simulink model "motorStyrning"  (R2020b)
settings: Solver=VariableStepAuto  StartTime=0.0  StopTime=0.1  RelTol=1e-3
model workspace (MAT data in the model file):
  intervall = 300
  intervall2 = 1
  intervall3 = 1
  timeTTT : Simulink.Signal (value not decoded)
libraries: fl_lib x116, ee_lib x24, nesl_utility x23
(part 2 of 2)

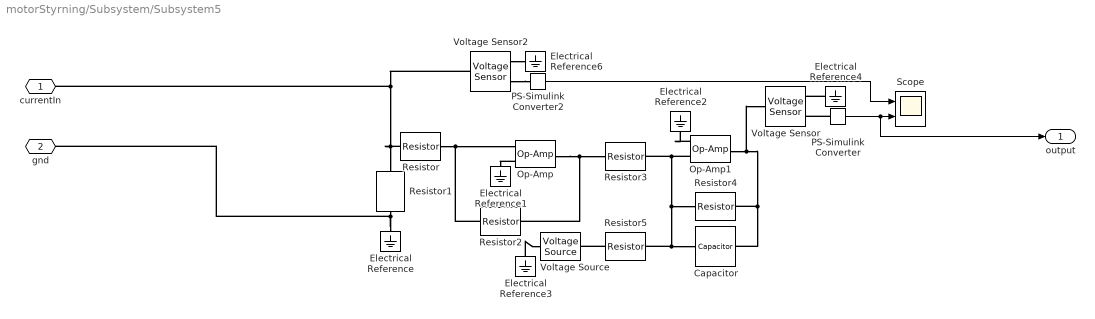
== system motorStyrning/Subsystem/Subsystem5 ==
  Capacitor : fl_lib/Electrical/Electrical Elements/Capacitor  c=10 nF  r=1e-6 Ohm  g=0 1/Ohm  i_specify=off  i_priority=None  i=0 A  i_nominal_specify=off  i_nominal_unit=A  i_nominal_value=1  v_specify=off  v_priority=None  v=0 V  v_nominal_specify=off  v_nominal_unit=V  v_nominal_value=1  vc_specify=off  vc_priority=High  vc=0 V  vc_nominal_specify=off  vc_nominal_unit=V  vc_nominal_value=1
  Electrical Reference{,1..4,6} (6 alike) : fl_lib/Electrical/Electrical Elements/Electrical Reference
  Op-Amp : fl_lib/Electrical/Electrical Elements/Op-Amp  outI_specify=off  outI_priority=None  outI=0 A  outI_nominal_specify=off  outI_nominal_unit=A  outI_nominal_value=1
  Op-Amp1 : fl_lib/Electrical/Electrical Elements/Op-Amp  outI_specify=off  outI_priority=None  outI=0 A  outI_nominal_specify=off  outI_nominal_unit=A  outI_nominal_value=1
  PS-Simulink Converter : nesl_utility/PS-Simulink Converter  PhysicalDomain=network_engine_domain  SubClassName=ps_output  LeftPortType=input  RightPortType=output  PseudoPeriodic=off  Frequencies=[]  Unit=inherit  AffineConversion=off
  PS-Simulink Converter2 : nesl_utility/PS-Simulink Converter  PhysicalDomain=network_engine_domain  SubClassName=ps_output  LeftPortType=input  RightPortType=output  PseudoPeriodic=off  Frequencies=[]  Unit=inherit  AffineConversion=off
  Resistor : fl_lib/Electrical/Electrical Elements/Resistor  R=10 kOhm  i_specify=off  i_priority=None  i=0 A  i_nominal_specify=off  i_nominal_unit=A  i_nominal_value=1  v_specify=off  v_priority=None  v=0 V  v_nominal_specify=off  v_nominal_unit=V  v_nominal_value=1
  Resistor1 : fl_lib/Electrical/Electrical Elements/Resistor  R=60 Ohm  i_specify=off  i_priority=None  i=0 A  i_nominal_specify=off  i_nominal_unit=A  i_nominal_value=1  v_specify=off  v_priority=None  v=0 V  v_nominal_specify=off  v_nominal_unit=V  v_nominal_value=1
  Resistor2 : fl_lib/Electrical/Electrical Elements/Resistor  R=8275 Ohm  i_specify=off  i_priority=None  i=0 A  i_nominal_specify=off  i_nominal_unit=A  i_nominal_value=1  v_specify=off  v_priority=None  v=0 V  v_nominal_specify=off  v_nominal_unit=V  v_nominal_value=1
  Resistor3 : fl_lib/Electrical/Electrical Elements/Resistor  R=10 kOhm  i_specify=off  i_priority=None  i=0 A  i_nominal_specify=off  i_nominal_unit=A  i_nominal_value=1  v_specify=off  v_priority=None  v=0 V  v_nominal_specify=off  v_nominal_unit=V  v_nominal_value=1
  Resistor4 : fl_lib/Electrical/Electrical Elements/Resistor  R=10 kOhm  i_specify=off  i_priority=None  i=0 A  i_nominal_specify=off  i_nominal_unit=A  i_nominal_value=1  v_specify=off  v_priority=None  v=0 V  v_nominal_specify=off  v_nominal_unit=V  v_nominal_value=1
  Resistor5 : fl_lib/Electrical/Electrical Elements/Resistor  R=29.7 kOhm  i_specify=off  i_priority=None  i=0 A  i_nominal_specify=off  i_nominal_unit=A  i_nominal_value=1  v_specify=off  v_priority=None  v=0 V  v_nominal_specify=off  v_nominal_unit=V  v_nominal_value=1
  Scope : Scope  NumInputPorts=2
  Voltage Sensor : fl_lib/Electrical/Electrical Sensors/Voltage Sensor
  Voltage Sensor2 : fl_lib/Electrical/Electrical Sensors/Voltage Sensor
  Voltage Source : ee_lib/Sources/Voltage Source  dc_voltage=-15 V  ac_voltage=0 V  ac_shift=0 rad  ac_frequency=60 Hz  noise_mode=0  PSD=0 V^2/Hz  repeatability=1  auto_seed=3243031446  user_seed=0  sample_time=1e-3 s  i_specify=off  i_priority=None  i=0 A  i_nominal_specify=off  i_nominal_unit=A  i_nominal_value=1  v_specify=off  v_priority=None  v=0 V  v_nominal_specify=off  v_nominal_unit=V  v_nominal_value=1
  currentIn : PMIOPort  Side=Left
  gnd : PMIOPort  Port=2  Side=Left
  output : Outport
  wires:
  PS-Simulink Converter/1 -> output/1, Scope/2
  PS-Simulink Converter2/1 -> Scope/1
  connections:
  Resistor1/RConn1 -- gnd/RConn1 -- Electrical Reference/LConn1
  Voltage Sensor2/RConn1 -- PS-Simulink Converter2/LConn1
  Voltage Sensor2/RConn2 -- Electrical Reference6/LConn1
  PS-Simulink Converter/LConn1 -- Voltage Sensor/RConn1
  Resistor5/LConn1 -- Voltage Source/LConn1
  Op-Amp/LConn2 -- Electrical Reference1/LConn1
  Op-Amp1/LConn2 -- Resistor3/RConn1 -- Resistor5/RConn1 -- Capacitor/LConn1 -- Resistor4/LConn1
  Electrical Reference3/LConn1 -- Voltage Source/RConn1
  Electrical Reference4/LConn1 -- Voltage Sensor/RConn2
  Op-Amp1/LConn1 -- Electrical Reference2/LConn1
  Capacitor/RConn1 -- Resistor4/RConn1 -- Op-Amp1/RConn1 -- Voltage Sensor/LConn1
  Op-Amp/RConn1 -- Resistor3/LConn1 -- Resistor2/RConn1
  Resistor/RConn1 -- Resistor2/LConn1 -- Op-Amp/LConn1
  Voltage Sensor2/LConn1 -- Resistor/LConn1 -- Resistor1/LConn1 -- currentIn/RConn1

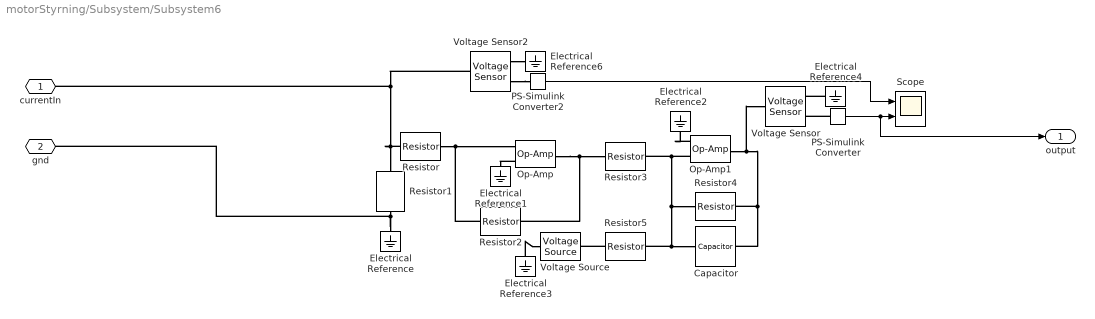
== system motorStyrning/Subsystem/Subsystem6 ==
  Capacitor : fl_lib/Electrical/Electrical Elements/Capacitor  c=10 nF  r=1e-6 Ohm  g=0 1/Ohm  i_specify=off  i_priority=None  i=0 A  i_nominal_specify=off  i_nominal_unit=A  i_nominal_value=1  v_specify=off  v_priority=None  v=0 V  v_nominal_specify=off  v_nominal_unit=V  v_nominal_value=1  vc_specify=off  vc_priority=High  vc=0 V  vc_nominal_specify=off  vc_nominal_unit=V  vc_nominal_value=1
  Electrical Reference{,1..4,6} (6 alike) : fl_lib/Electrical/Electrical Elements/Electrical Reference
  Op-Amp : fl_lib/Electrical/Electrical Elements/Op-Amp  outI_specify=off  outI_priority=None  outI=0 A  outI_nominal_specify=off  outI_nominal_unit=A  outI_nominal_value=1
  Op-Amp1 : fl_lib/Electrical/Electrical Elements/Op-Amp  outI_specify=off  outI_priority=None  outI=0 A  outI_nominal_specify=off  outI_nominal_unit=A  outI_nominal_value=1
  PS-Simulink Converter : nesl_utility/PS-Simulink Converter  PhysicalDomain=network_engine_domain  SubClassName=ps_output  LeftPortType=input  RightPortType=output  PseudoPeriodic=off  Frequencies=[]  Unit=inherit  AffineConversion=off
  PS-Simulink Converter2 : nesl_utility/PS-Simulink Converter  PhysicalDomain=network_engine_domain  SubClassName=ps_output  LeftPortType=input  RightPortType=output  PseudoPeriodic=off  Frequencies=[]  Unit=inherit  AffineConversion=off
  Resistor : fl_lib/Electrical/Electrical Elements/Resistor  R=10 kOhm  i_specify=off  i_priority=None  i=0 A  i_nominal_specify=off  i_nominal_unit=A  i_nominal_value=1  v_specify=off  v_priority=None  v=0 V  v_nominal_specify=off  v_nominal_unit=V  v_nominal_value=1
  Resistor1 : fl_lib/Electrical/Electrical Elements/Resistor  R=60 Ohm  i_specify=off  i_priority=None  i=0 A  i_nominal_specify=off  i_nominal_unit=A  i_nominal_value=1  v_specify=off  v_priority=None  v=0 V  v_nominal_specify=off  v_nominal_unit=V  v_nominal_value=1
  Resistor2 : fl_lib/Electrical/Electrical Elements/Resistor  R=8275 Ohm  i_specify=off  i_priority=None  i=0 A  i_nominal_specify=off  i_nominal_unit=A  i_nominal_value=1  v_specify=off  v_priority=None  v=0 V  v_nominal_specify=off  v_nominal_unit=V  v_nominal_value=1
  Resistor3 : fl_lib/Electrical/Electrical Elements/Resistor  R=10 kOhm  i_specify=off  i_priority=None  i=0 A  i_nominal_specify=off  i_nominal_unit=A  i_nominal_value=1  v_specify=off  v_priority=None  v=0 V  v_nominal_specify=off  v_nominal_unit=V  v_nominal_value=1
  Resistor4 : fl_lib/Electrical/Electrical Elements/Resistor  R=10 kOhm  i_specify=off  i_priority=None  i=0 A  i_nominal_specify=off  i_nominal_unit=A  i_nominal_value=1  v_specify=off  v_priority=None  v=0 V  v_nominal_specify=off  v_nominal_unit=V  v_nominal_value=1
  Resistor5 : fl_lib/Electrical/Electrical Elements/Resistor  R=29.7 kOhm  i_specify=off  i_priority=None  i=0 A  i_nominal_specify=off  i_nominal_unit=A  i_nominal_value=1  v_specify=off  v_priority=None  v=0 V  v_nominal_specify=off  v_nominal_unit=V  v_nominal_value=1
  Scope : Scope  NumInputPorts=2
  Voltage Sensor : fl_lib/Electrical/Electrical Sensors/Voltage Sensor
  Voltage Sensor2 : fl_lib/Electrical/Electrical Sensors/Voltage Sensor
  Voltage Source : ee_lib/Sources/Voltage Source  dc_voltage=-15 V  ac_voltage=0 V  ac_shift=0 rad  ac_frequency=60 Hz  noise_mode=0  PSD=0 V^2/Hz  repeatability=1  auto_seed=4112460543  user_seed=0  sample_time=1e-3 s  i_specify=off  i_priority=None  i=0 A  i_nominal_specify=off  i_nominal_unit=A  i_nominal_value=1  v_specify=off  v_priority=None  v=0 V  v_nominal_specify=off  v_nominal_unit=V  v_nominal_value=1
  currentIn : PMIOPort  Side=Left
  gnd : PMIOPort  Port=2  Side=Left
  output : Outport
  wires:
  PS-Simulink Converter/1 -> output/1, Scope/2
  PS-Simulink Converter2/1 -> Scope/1
  connections:
  Resistor1/RConn1 -- Electrical Reference/LConn1 -- gnd/RConn1
  Voltage Sensor2/RConn1 -- PS-Simulink Converter2/LConn1
  Voltage Sensor2/RConn2 -- Electrical Reference6/LConn1
  PS-Simulink Converter/LConn1 -- Voltage Sensor/RConn1
  Resistor5/LConn1 -- Voltage Source/LConn1
  Op-Amp/LConn2 -- Electrical Reference1/LConn1
  Op-Amp1/LConn2 -- Resistor3/RConn1 -- Resistor5/RConn1 -- Capacitor/LConn1 -- Resistor4/LConn1
  Electrical Reference3/LConn1 -- Voltage Source/RConn1
  Electrical Reference4/LConn1 -- Voltage Sensor/RConn2
  Op-Amp1/LConn1 -- Electrical Reference2/LConn1
  Capacitor/RConn1 -- Resistor4/RConn1 -- Op-Amp1/RConn1 -- Voltage Sensor/LConn1
  Op-Amp/RConn1 -- Resistor3/LConn1 -- Resistor2/RConn1
  Resistor/RConn1 -- Resistor2/LConn1 -- Op-Amp/LConn1
  Voltage Sensor2/LConn1 -- Resistor/LConn1 -- Resistor1/LConn1 -- currentIn/RConn1

== matlab function motorStyrning/Subsystem/MATLAB Function ==
  data: freeW input; u input; y output
function y = fcn(freeW, u)
%#codegen
if u == 2
    
    if freeW==0
    a0 = 0; a1 = 0; a2 = 10; b0 = 10; b1 = 0; b2 = 10;  %% a2 var 10 innan AW ändrade
    else
    a0 = 0; a1 = 0; a2 = 10; b0 = 0; b1 = 0; b2 = 10;   %% a2 var 10 innan AW ändrade
    end
    
elseif u == 10 || 32
    
    if freeW == 0
      a0 = 0; a1 = 10; a2 = 0; b0 = 10; b1 = 10; b2 = 0;  
    else
        a0 = 0; a1 = 10; a2 = 0; b0 = 0; b1 = 10; b2 = 0;
    end
elseif u == 20
        
    if freeW == 0
        a0 = 10; a1 = 0; a2 = 0; b0 = 10; b1 = 0; b2 = 10;
    else
       a0 = 10; a1 = 0; a2 = 0; b0 = 10; b1 = 0; b2 = 0; 
    end
elseif u == 12
        
    if freeW == 0
        a0 = 0; a1 = 0; a2 = 10; b0 = 10; b1 = 0; b2 = 10;
    else
        a0 = 0; a1 = 0; a2 = 0; b0 = 10; b1 = 0; b2 = 0;
    end
elseif u == 30
        
    if freeW == 0
        a0 = 0; a1 = 10; a2 = 0; b0 = 0; b1 = 10; b2 = 10;
    else
        a0 = 0; a1 = 0; a2 = 0; b0 = 0; b1 = 0; b2 = 10;
    end
elseif u == 22
        
    if freeW == 0
        a0 = 10; a1 = 0; a2 = 0; b0 = 10; b1 = 10; b2 = 0;
    else
        a0 = 0; a1 = 0; a2 = 0; b0 = 10; b1 = 0; b2 = 0;
    end
end

A = [a0,a1,a2,b0,b1,b2]';

y = A;

== matlab function motorStyrning/Subsystem/MATLAB Function2 ==
  data: u2 input; u1 input; u input; y output
function y = fcn(u2, u1, u)

A = [u,u1,u2]';

for n = 1 : length(A)
    A(n) = abs(A(n) * 50 - 250);
    if A(n) <= 251
         A(n) = 0;
    else
         A(n) = 1;
    end
end

if sum(A) > 0
    y = 1;
else
    y = 0;
end

== matlab function motorStyrning/Subsystem/MATLAB Function1 ==
  data: freeW input; u input; y output
function y = fcn(freeW, u)
%#codegen
%if u == 2
    %a0 = 0; a1 = 10; a2 = 10; b0 = 0; b1 = 10; b2 = 10;
%elseif u == 10 || 32
       % a0 = 0; a1 = 10; a2 = 0; b0 = 10; b1 = 10; b2 = 0;
%elseif u == 20
       % a0 = 10; a1 = 0; a2 = 0; b0 = 0; b1 = 10; b2 = 10;
%elseif u == 12
      %  a0 = 0; a1 = 00; a2 = 10; b0 = 10; b1 = 0; b2 = 10;
%elseif u == 30
      %  a0 = 0; a1 = 10; a2 = 0; b0 = 0; b1 = 10; b2 = 10;
%elseif u == 22
       % a0 = 10; a1 = 00; a2 = 0; b0 = 10; b1 = 10; b2 = 0;
%end

if u == 2
    
    if freeW==0
        t0 = 0; t1 = 0; t2 = 10; t3 = 0; t4 = 10; t5 = 0;  
    else
        t0 = 0; t1 = 0; t2 = 10; t3 = 0; t4 = 0; t5 = 0;  
    end
    
elseif u == 10 || 32
    
    if freeW == 0
         t0 = 0; t1 = 10; t2 = 0; t3 = 10; t4 = 0; t5 = 0;  
    else
         t0 = 0; t1 = 0; t2 = 0; t3 = 0; t4 = 0; t5 = 0;
    end
    
elseif u == 20
    
    if freeW == 0
        t0 = 10; t1 = 0; t2 = 0; t3 = 10; t4 = 0; t5 = 10;  
    else
        t0 = 0; t1 = 0; t2 = 0; t3 = 0; t4 = 0; t5 = 10;
    end
    
elseif u == 12
    
    if freeW == 0
        t0 = 0; t1 = 0; t2 = 10; t3 = 10; t4 = 0; t5 = 0;  
    else
        t0 = 0; t1 = 0; t2 = 10; t3 = 0; t4 = 0; t5 = 0;
    end
    
elseif u == 30
    
    if freeW == 0
        t0 = 0; t1 = 10; t2 = 0; t3 = 0; t4 = 0; t5 = 10;  
    else
        t0 = 0; t1 = 10; t2 = 0; t3 = 0; t4 = 0; t5 = 0;
    end
    
elseif u == 22
    
    if freeW == 0
        t0 = 10; t1 = 0; t2 = 0; t3 = 0; t4 = 10; t5 = 0;  
    else
        t0 = 0; t1 = 0; t2 = 0; t3 = 0; t4 = 10; t5 = 0;
    end
end
    
    
A = [t0,t1,t2,t3,t4,t5]';
%if freeW >= 1
   % for n = 1 : length(A)
    %  if sum(A) > 10
     %     A(n) = 0;
     % end
  %  end
%end
y = A;
